simulink model "RCcircuit"  (R2020a)
settings: Solver=VariableStepAuto  StartTime=0.0  StopTime=10.0  RelTol=1e-3
PostLoadFcn:
  | R=10;
  | C=10e-6;
undefined symbols (not defined in the file or in its folder): init
settings Model: DataDictionary=DataDiction.sldd  Creator=Hp  LastModifiedBy=Hp
settings DataIOCC: ExternalInput=init

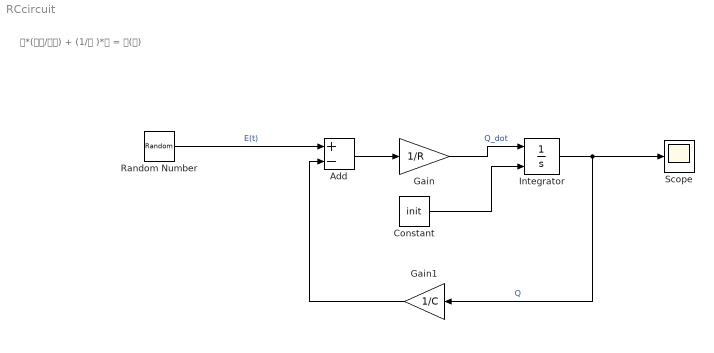
== system RCcircuit ==
  note: 𝑅*(𝑑𝑄/𝑑𝑡) + (1/𝐶 )*𝑄 = 𝐸(𝑡)
  Add : Sum  Inputs=+-
  Constant : Constant  Value=init
  Gain : Gain  Gain=1/R
  Gain1 : Gain  Gain=1/C
  Integrator : Integrator  InitialConditionSource=external
  Random Number : RandomNumber  SampleTime=0.1
  Scope : Scope
  wires:
  Integrator/1 -> Scope/1, Gain1/1  "Q"
  Gain/1 -> Integrator/1  "Q_dot"
  Random Number/1 -> Add/1  "E(t)"
  Add/1 -> Gain/1
  Gain1/1 -> Add/2
  Constant/1 -> Integrator/2
